simulink model "func2_d"  (R2024a)
settings: Solver=VariableStepAuto  StartTime=0.0  StopTime=10.0  RelTol=1e-3  EnableMultiTasking=on
libraries: vmcUtilities x2, hlsBasic x1, fixedpoint_complex_2_lib x1
settings Model: Creator=abehbood  LastModifiedBy=robg
settings SolverCC: AlgebraicLoopSolver=TrustRegion
settings DataIOCC: ReturnWorkspaceOutputs=off
settings OptimizationCC: LifeSpan=inf
settings DebuggingCC: UnconnectedInputMsg=warning  UnconnectedOutputMsg=warning  UnconnectedLineMsg=warning  SFUnexpectedBacktrackingDiag=warning  SFNoUnconditionalDefaultTransitionDiag=warning  ArithmeticOperatorsInVariantConditions=warning
settings ModelReferenceCC: EnableRefExpFcnMdlSchedulingChecks=on
settings SFSimCC: SimUseLocalCustomCode=off  CustomCodeUndefinedFunction=UseInterfaceOnly
settings RTWCC: RTWUseLocalCustomCode=off  GPUComputeCapability=3.5  DLArmComputeVersion=19.05
settings CodeAppCC: StateflowObjectComments=on
settings GRTTargetCC: TargetLangStandard=C89/C90 (ANSI)
settings ConfigComp: CovMetricSettings=dw  CovSaveCumulativeToWorkspaceVar=on  CovSaveSingleToWorkspaceVar=on  CovExternalEMLEnable=off  CovBoundaryAbsTol=1.0e-5

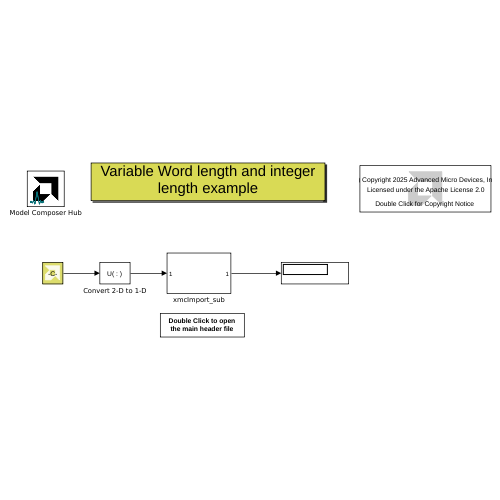
[thumbnail: Simulink's stored preview of the top-level diagram]
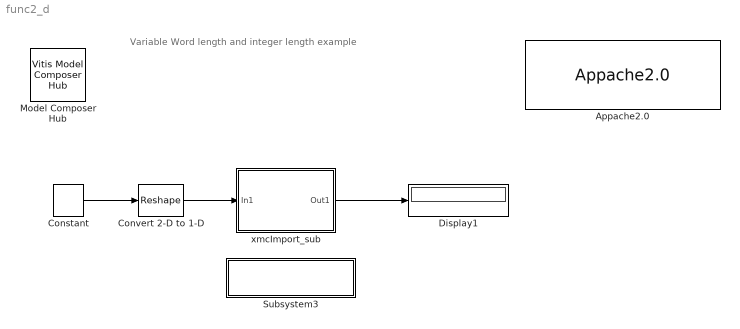
== system func2_d ==
  note: Variable Word length and integer length example
  Appache2.0 : vmcUtilities/Appache2.0
  Constant : hlsBasic/Constant  Value=[1 2 3 4 5 6]  VectorParams1D=off  SampleTime=1.0  OutDataType=fixed  TypeExp=''  Signedness=Signed  WordLength=16  FractionalLength=5  RoundingMode=Truncation to minus infinity  OverflowMode=Wrap around
  Convert 2-D to 1-D : Reshape
  Display1 : Display
  Model Composer Hub : vmcUtilities/Vitis Model Composer Hub  Tag=genX  CodeGeneration=off  SubsystemName=xmcImport_sub  StartColumn=1  NumberOfColumns=1  TargetDirectory=./code  exportDesign=off  analyzeDesign=off  validateDesignOnHw=off  ExportType=IP Catalog  IpVendor=xilinx.com  IpLibrary=hls  IpVersion=1.0  IpHWLanguage=Verilog  AieCompilerOptions={}  AieSimulatorOptions={}  CreateTestbench=off  TestbenchStackSize=10  RunRtlSim=off  RunCSim=off  RunAieSim=off  AieSimTimeout=50000  RunAieSimProfiling=off  LaunchVitisAnalyzer=off  PlotOutput=off  RunX86Sim=off  X86SimTimeout=10  GenHwImage=off  GenLibadfXo=off  GenHwValidationCode=off  PlatformType=Not Specified  HwSystemType=Baremetal  HwValidationTarget=hw  ProjDevice=xcku11p-ffva1156-1-e  ProjDevicePart=xcku11p-ffva1156-1-e  SamplePeriod=-1  ClockFrequency=200  DataPathParallelism=1  xilinxfamily=Kintex7  part=xc7k325t  speed=-3  package=fbg676  directory=./netlist  testbench=off  incr_netlist=off  synthesis_tool=Vivado  clock_wrapper=Clock Enables  dbl_ovrd=According to Block Masks  dcm_input_clock_period=10  sysclk_period=10  simulink_period=1  eval_field=0  LogFileName=''  NThreads=4
  Subsystem3 : Subsystem
      settings: OpenFcn=xmcOpenFileEx
      mask Display: disp(sprintf('Double Click to open\nthe main header file'))
  xmcImport_sub : Subsystem
  wires:
  Constant/1 -> Convert 2-D to 1-D/1
  Convert 2-D to 1-D/1 -> xmcImport_sub/1(In1)
  xmcImport_sub/1(Out1) -> Display1/1

== system func2_d/Subsystem3 ==

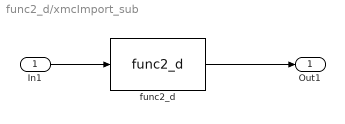
== system func2_d/xmcImport_sub ==
  In1 : Inport
  func2_d : fixedpoint_complex_2_lib/func2_d  LibraryFunction=func2_d  IncludeFiles={'func2_d.h'}  SourceFiles={}  IncludeDirectories={}  TemplateParams={'int WordLen'; 'int IntLen'; 'int SIZE'}  FunctionParamTypes={xmcDataType('void'); xmcDataType('const ap_fixed<WordLen, IntLen>'); xmcDataType('ap_fixed<WordLen + 1, IntLen> &')}  FunctionParamPassbys={0.000000000000000000e+00; 0.000000000000000000e+00; 1.000000000000000000e+00}  FunctionParamDimensions={'1'; '[SIZE]'; '1'}  FunctionParamNames={'return'; 'in1'; 'out'}  FunctionParamDir={0.000000000000000000e+00; 1.000000000000000000e+00; 2.000000000000000000e+00}  FunctionParamSupportsStreaming={false; false; false}  BufferDepth={'0'}  FunctionParamValues={'0'; '0'; '0'}  ThroughputFactors={''}
  Out1 : Outport
  wires:
  func2_d/1 -> Out1/1
  In1/1 -> func2_d/1
